simulink model "MISSIONSTEP"  (R2022b)
settings: Solver=VariableStepAuto  StartTime=0.0  StopTime=10.0  RelTol=1e-3
settings Model: Creator=lucaerviati  LastModifiedBy=lucaerviati
settings DataIOCC: SaveOutput=off  SaveTime=off
settings GRTTargetCC: CombineOutputUpdateFcns=off  MatFileLogging=off

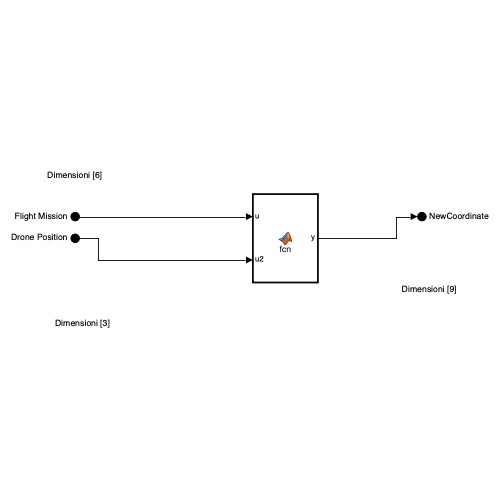
[thumbnail: Simulink's stored preview of the top-level diagram]
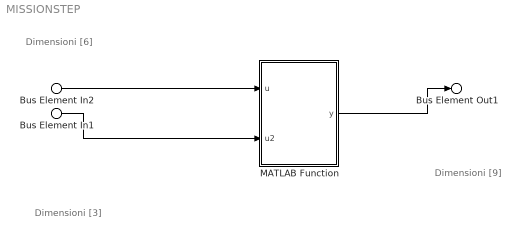
== system MISSIONSTEP ==
  note: Dimensioni [9]
  note: Dimensioni [3]
  note: Dimensioni [6]
  Bus Element In2 : Inport  PortName=Flight Mission
  Bus Element In1 : Inport  Port=2  PortName=Drone Position
  MATLAB Function : MATLAB Function  TreatAsAtomicUnit=on
  Bus Element Out1 : Outport  PortName=NewCoordinate
  wires:
  Bus Element In2/1 -> MATLAB Function/1(u)
  MATLAB Function/1(y) -> Bus Element Out1/1
  Bus Element In1/1 -> MATLAB Function/2(u2)

== matlab function MISSIONSTEP/MATLAB Function ==
  data: u input; y output; u2 input
function y = fcn(u,u2)

u = 1;
if u>0
    y = [1,3,30,4,1,1,12,3,4];
else
    y = [0,3,30,4,1,1,12,3,4];
end
